simulink model "modal2"  (R2018b)
settings: Solver=VariableStepAuto  StartTime=0.0  StopTime=10.0  MaxStep=0.01  RelTol=1e-3
InitFcn:
  | A = [0 1; 4 0];
  | B = [1; 1];
  | C = [3 0];
  | D = 3;
  | K = [3.4074 7.2593];
Description:
  | A = [0 1; 4 0];
  | B = [1; 1];
  | C = [3 0];
  | D = 3;
  | K = [3.4074 7.2593];
settings Model: Creator=kekos  LastModifiedBy=kekos

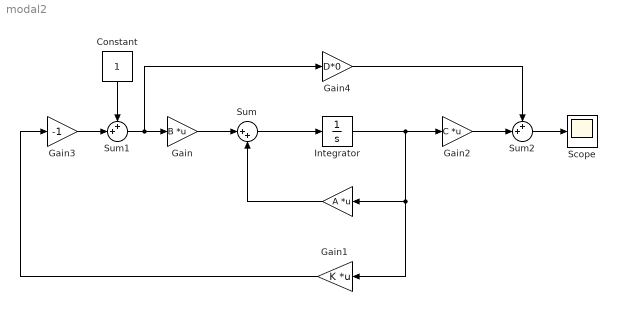
== system modal2 ==
  " " : Gain  Gain=A  Multiplication=Matrix(K*u)
  Constant : Constant
  Gain : Gain  Gain=B  Multiplication=Matrix(K*u)
  Gain1 : Gain  Gain=K  Multiplication=Matrix(K*u)
  Gain2 : Gain  Gain=C  Multiplication=Matrix(K*u)
  Gain3 : Gain  Gain=-1
  Gain4 : Gain  Gain=D*0
  Integrator : Integrator
  Scope : Scope
  Sum : Sum  Inputs=|++
  Sum1 : Sum  Inputs=++|
  Sum2 : Sum  Inputs=++|
  wires:
  Sum/1 -> Integrator/1
  Integrator/1 -> Gain2/1, Gain1/1, " "/1
  " "/1 -> Sum/2
  Gain/1 -> Sum/1
  Sum1/1 -> Gain4/1, Gain/1
  Constant/1 -> Sum1/1
  Gain1/1 -> Gain3/1
  Gain2/1 -> Sum2/2
  Gain3/1 -> Sum1/2
  Gain4/1 -> Sum2/1
  Sum2/1 -> Scope/1
